simulink library "NREL_Diesel_Genset_lib"  (Simulink 8.1)
settings: Solver=ode45  StartTime=0.0  StopTime=10.0  RelTol=1e-3
values from neighbouring files (symbols this model uses):
  T3dend = [ 1.0000   -0.9913 ]    [initGTS.m]
  T3numd = [ 0    0.0087 ]    [initGTS.m]
  T4numd = [ 27.7778  -27.7237 ]    [initGTS.m]
undefined symbols (not defined in the file or in its folder): DiscIntNeverNeededParam, Efd0, Efd1, Efd2, GP, Ka, Ke, Kf, SeEfd1, SeEfd2, Ta, Te, Tf, Ts, VR0, VRmax, VRmin
libraries: simulink x17, powerlib x9, powerlib_extras x2, powerlib_models x1
(part 1 of 2)
settings Model: Creator=ed12083  LastModifiedBy=pkoralew

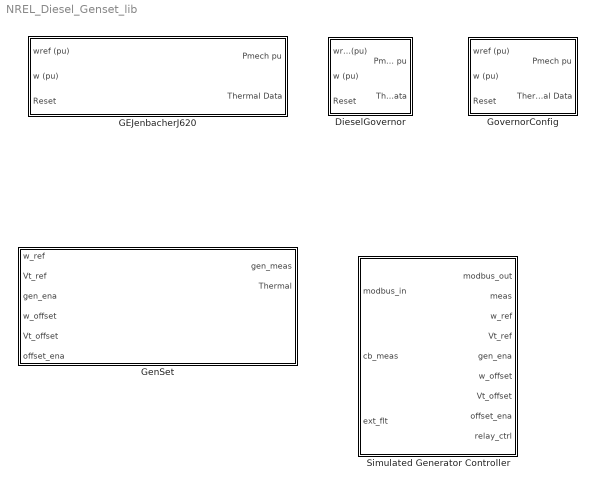
== system NREL_Diesel_Genset_lib ==
  DieselGovernor : Subsystem  mask(Diesel Engine & Governor){K=GP.Gov.Kp, Ta=[0.025 0.0009 0.00574], Tlim=[0 2], Td=0.024, Pm0=0.00005}
      mask prompts: K "Regulator gain K:"; Ta "Actuator time constants [T4 T5 T6] (s) :"; Tlim "Torque limits [Tmin Tmax] (pu) :"; Td "Engine time delay Td (s) :"; Pm0 "Initial value of mechanical power  Pm0 (pu) :"
      mask help:
      | This block implements a diesel engine and governor system:
      | 1st and 2nd inputs: Desired and actual speed (pu)
      | Output: Diesel engine mechanical power.Motor inertia should be combined with generator.
      |
      | Actuator transfer function :
      |      Ha= (1+T4.s) / [ (s (1+T5.s)(1+T6.s) ]
      | Motor :
      |      Time delay Td
      |
      | (See reference in Tutorial Session 5)
  GEJenbacherJ620 : Subsystem  mask{cd=.8, H=47133, keq=1.3962, Ma=.029, Meq=.0285, Mf=.019, P0=800000, Pm=37241, R=8.314, T0=300, Tm=325, thermalEfficiency=.45, V=0.031, Vd=0.125, volumeEfficiency=.9, P=3, I=3, UL=1.05, LL=0, UPL=1.5, LPL=0}
      mask prompts: cd "Discharge coefficient - cd"; H "NG heating value - H"; keq "Equivalent ratio of specific heats of air/fuel mixture - keq"; Ma "Molecular weight of air - Ma"; Meq "Equivalent molecular weight of air/fuel mixture - Meq"; Mf "Molecular weight of NG - Mf"; P0 "Throttle inlet air pressure - P0"; Pm "Intake manifold pressure - Pm"; R "Universal gas constant - R"; T0 "Throttle inlet charge temperature - T0"; Tm "Intake manifold temperature - Tm"; thermalEfficiency "Thermal efficiency - thermalEfficiency"; V "Manifold plus port passage volume - V"; Vd "Engine displacement - Vd"; volumeEfficiency "Volumetric efficiency - volumeEfficiency"; P "Proportional Gain - P"; I "Integral Gain - I"; UL "Upper Integrator Limit - UL"; LL "Lower Integrator Limit - LL"; UPL "Upper Power Limit - UPL"; LPL "Lower Power Limit - LPL"
      mask help: All units are MKS. Refer to "Modeling and Validation of a Lean Burn Natural Gas Engine", Gangopadhyay et. al., ASME 2001
  GenSet : Subsystem  mask{GenSel=3.5MVA natural gas generator}
      mask prompts: GenSel "Generator Preset"
      mask init:
      | GP = initDiesel(GenSel);
      | 
      | dispstr = 'Diesel Generator\n';
      | dispstr = [dispstr 'Pn=' num2str(GP.Pn/1000) ' kW\n'];
      | dispstr = [dispstr 'Vn=' num2str(GP.Vn/1000) ' kV\n'];
      | 
      | govPath = [gcb '/GeneratorWPrimaryControllers/DieselSpeed&Voltage/Governor'];
      | 
      | switch GenSel
      |     case 1
      |         set_param(govPath, 'BlockChoice', 'DieselGovernor');
      |     case 2
      |         set_param(govPath, 'BlockChoice', 'DieselGovernor');
      |     case 3
      |         set_param(govPath, 'BlockChoice', 'DieselGovernor');
      |         %set_param(govPath, 'BlockChoice', 'GEJenbacherJ620');
      | end
      mask TypeOptions GenSel: 4MVA diesel generator | 80kVA diesel generator | 3.5MVA natural gas generator
      mask Display: disp(dispstr);
  GovernorConfig : Subsystem  BlockChoice=DieselGovernor
      settings: TemplateBlock=self  MemberBlocks=DieselGovernor,GEJenbacherJ620
  Simulated Generator Controller : Subsystem  mask{GenSel=80kVA diesel generator}
      mask prompts: GenSel "Generator preset"
      mask init:
      | GP = initGensetCtrl(GenSel);
      | 
      | dispstr = 'Generator controller\n';
      | dispstr = [dispstr 'Pn=' num2str(GP.Pn/1000) ' kW\n'];
      | dispstr = [dispstr 'Vn=' num2str(GP.Vn/1000) ' kV\n'];
      mask TypeOptions GenSel: 4MVA diesel generator | 80kVA diesel generator | 3.5MVA natural gas generator
      mask Display: disp(dispstr);

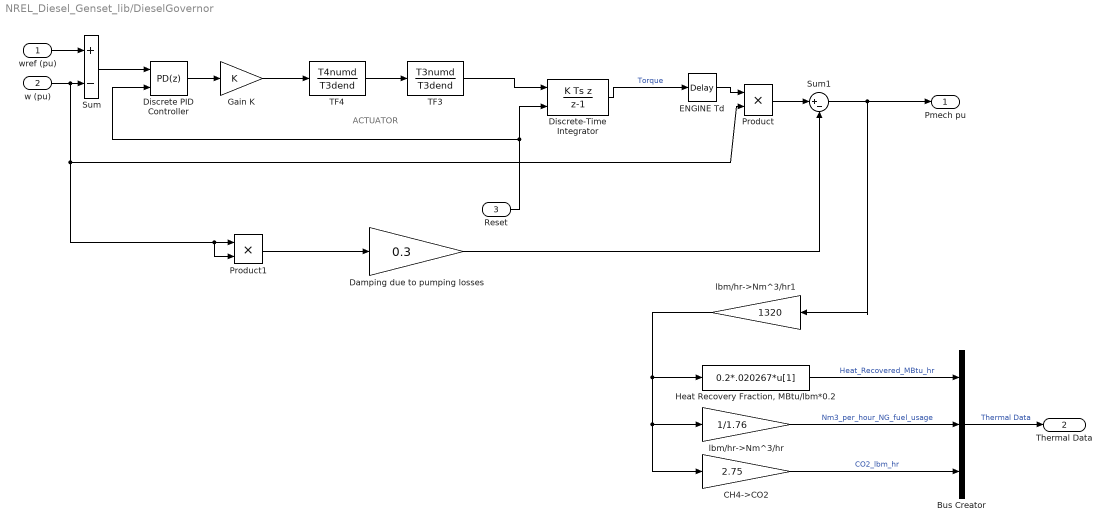
== system NREL_Diesel_Genset_lib/DieselGovernor ==
  note: ACTUATOR
  wref (pu) : Inport
  w (pu) : Inport  Port=2
  Reset : Inport  Port=3
  Bus Creator : BusCreator  Inputs=3
  CH4->CO2 : Gain  Gain=2.75
  Damping due to pumping losses : Gain  Gain=0.3
  Discrete PID Controller : simulink/Continuous/PID Controller  Controller=PD  TimeDomain=Discrete-time  SampleTime=-1  IntegratorMethod=Forward Euler  FilterMethod=Forward Euler  Form=Parallel  P=1  I=0  D=0.5  N=10000  InitialConditionSource=internal  InitialConditionForIntegrator=0  InitialConditionForFilter=0  ExternalReset=level  ZeroCross=off  LimitOutput=off  UpperSaturationLimit=.5  LowerSaturationLimit=-.5  LinearizeAsGain=off  AntiWindupMode=none  Kb=1  TrackingMode=off  Kt=1  PParamMin=[]  PParamMax=[]  IParamMin=[]  IParamMax=[]  DParamMin=[]  DParamMax=[]  NParamMin=[]  NParamMax=[]  KbParamMin=[]  KbParamMax=[]  KtParamMin=[]  KtParamMax=[]  POutMin=[]  POutMax=[]  IOutMin=[]  IOutMax=[]  DOutMin=[]  DOutMax=[]  NOutMin=[]  NOutMax=[]  KbOutMin=[]  KbOutMax=[]  KtOutMin=[]  KtOutMax=[]  IntegratorOutMin=[]  IntegratorOutMax=[]  FilterOutMin=[]  FilterOutMax=[]  SumOutMin=[]  SumOutMax=[]  SumI1OutMin=[]  SumI1OutMax=[]  SumI2OutMin=[]  SumI2OutMax=[]  SumI3OutMin=[]  SumI3OutMax=[]  SumDOutMin=[]  SumDOutMax=[]  SaturationOutMin=[]  SaturationOutMax=[]  IntegratorContinuousStateAttributes=''  IntegratorStateMustResolveToSignalObject=off  IntegratorRTWStateStorageClass=Auto  FilterContinuousStateAttributes=''  FilterStateMustResolveToSignalObject=off  FilterRTWStateStorageClass=Auto
  Discrete-Time Integrator : DiscreteIntegrator  IntegratorMethod=Integration: Backward Euler  ExternalReset=level  InitialCondition=Pm0  SampleTime=-1  LimitOutput=on  UpperSaturationLimit=Tlim(2)  LowerSaturationLimit=Tlim(1)  ICPrevOutput=DiscIntNeverNeededParam  ICPrevScaledInput=DiscIntNeverNeededParam
  ENGINE Td : TransportDelay  DelayTime=Td  InitialOutput=Pm0  BufferSize=7168
  Gain K : Gain  Gain=K  SaturateOnIntegerOverflow=on  OutDataTypeStr=Inherit: Same as input  ParamDataTypeStr=Inherit: Same as input
  "Heat Recovery Fraction, MBtu/lbm*0.2 " : Fcn  Expr=0.2*.020267*u[1]
  Product : Product  SaturateOnIntegerOverflow=on  InputSameDT=on  OutDataTypeStr=Inherit: Same as first input
  Product1 : Product
  Sum : Sum  Inputs=+-  SaturateOnIntegerOverflow=on  InputSameDT=on  OutDataTypeStr=Inherit: Same as first input
  Sum1 : Sum  Inputs=|+-
  TF3 : DiscreteTransferFcn  Numerator=T3numd  Denominator=T3dend  SampleTime=Ts  RndMeth=Nearest
  TF4 : DiscreteTransferFcn  Numerator=T4numd  Denominator=T3dend  SampleTime=Ts
  lbm/hr->Nm^3/hr : Gain  Gain=1/1.76
  lbm/hr->Nm^3/hr1 : Gain  Gain=1320
  Pmech pu : Outport
  Thermal Data : Outport  Port=2
  wires:
  Reset/1 -> Discrete PID Controller/2, Discrete-Time Integrator/2
  TF4/1 -> TF3/1
  TF3/1 -> Discrete-Time Integrator/1
  Discrete-Time Integrator/1 -> ENGINE Td/1  "Torque"
  Product/1 -> Sum1/1
  wref (pu)/1 -> Sum/1
  ENGINE Td/1 -> Product/1
  Gain K/1 -> TF4/1
  Sum/1 -> Discrete PID Controller/1
  Discrete PID Controller/1 -> Gain K/1
  w (pu)/1 -> Sum/2, Product1/1, Product1/2, Product/2
  Product1/1 -> Damping due to pumping losses/1
  Sum1/1 -> Pmech pu/1, lbm/hr->Nm^3/hr1/1
  CH4->CO2/1 -> Bus Creator/3  "CO2_lbm_hr"
  lbm/hr->Nm^3/hr/1 -> Bus Creator/2  "Nm3_per_hour_NG_fuel_usage"
  "Heat Recovery Fraction, MBtu/lbm*0.2 "/1 -> Bus Creator/1  "Heat_Recovered_MBtu_hr"
  Damping due to pumping losses/1 -> Sum1/2
  Bus Creator/1 -> Thermal Data/1  "Thermal Data"
  lbm/hr->Nm^3/hr1/1 -> CH4->CO2/1, lbm/hr->Nm^3/hr/1, "Heat Recovery Fraction, MBtu/lbm*0.2 "/1

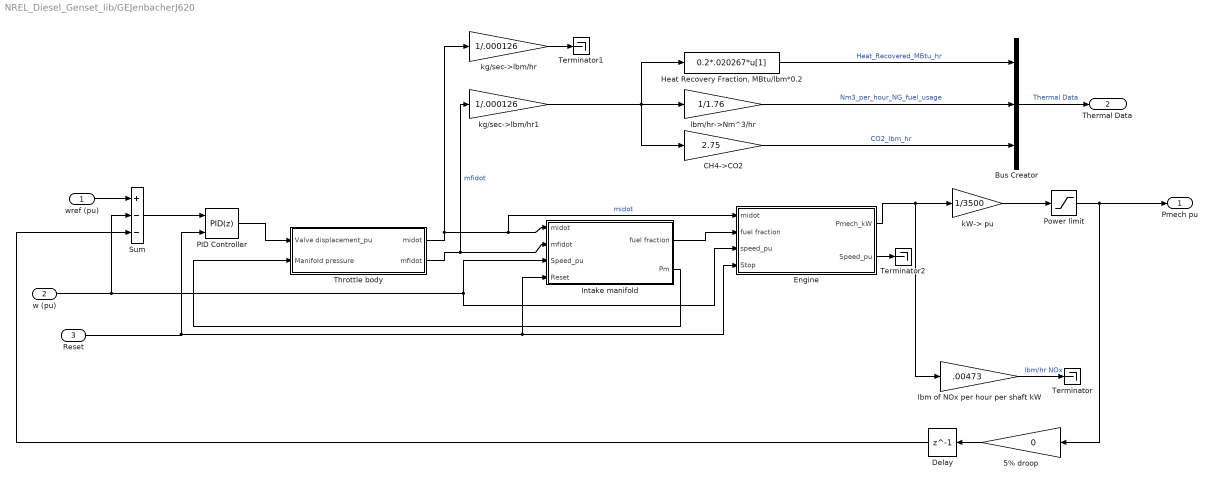
== system NREL_Diesel_Genset_lib/GEJenbacherJ620 ==
  wref (pu) : Inport
  w (pu) : Inport  Port=2
  Reset : Inport  Port=3
  5% droop : Gain  Gain=0
  Bus Creator : BusCreator  Inputs=3
  CH4->CO2 : Gain  Gain=2.75
  Delay : Delay  DelayLength=1  InitialCondition=0
  Engine : Subsystem
  "Heat Recovery Fraction, MBtu/lbm*0.2 " : Fcn  Expr=0.2*.020267*u[1]
  Intake manifold : Subsystem
  PID Controller : simulink/Continuous/PID Controller  Controller=PID  TimeDomain=Discrete-time  SampleTime=Ts  IntegratorMethod=Forward Euler  FilterMethod=Forward Euler  Form=Parallel  P=P  I=I  D=0  N=100  InitialConditionSource=internal  InitialConditionForIntegrator=0  InitialConditionForFilter=0  ExternalReset=level  LimitOutput=off  UpperSaturationLimit=inf  LowerSaturationLimit=-inf  LinearizeAsGain=on  AntiWindupMode=none  Kb=1  TrackingMode=off  Kt=1  PParamMin=[]  PParamMax=[]  IParamMin=[]  IParamMax=[]  DParamMin=[]  DParamMax=[]  NParamMin=[]  NParamMax=[]  KbParamMin=[]  KbParamMax=[]  KtParamMin=[]  KtParamMax=[]  POutMin=[]  POutMax=[]  IOutMin=[]  IOutMax=[]  DOutMin=[]  DOutMax=[]  NOutMin=[]  NOutMax=[]  KbOutMin=[]  KbOutMax=[]  KtOutMin=[]  KtOutMax=[]  IntegratorOutMin=[]  IntegratorOutMax=[]  FilterOutMin=[]  FilterOutMax=[]  SumOutMin=[]  SumOutMax=[]  SumI1OutMin=[]  SumI1OutMax=[]  SumI2OutMin=[]  SumI2OutMax=[]  SumI3OutMin=[]  SumI3OutMax=[]  SumDOutMin=[]  SumDOutMax=[]  SaturationOutMin=[]  SaturationOutMax=[]  IntegratorContinuousStateAttributes=''  IntegratorStateMustResolveToSignalObject=off  IntegratorRTWStateStorageClass=Auto  FilterContinuousStateAttributes=''  FilterStateMustResolveToSignalObject=off  FilterRTWStateStorageClass=Auto
  Power limit : Saturate  UpperLimit=UPL  LowerLimit=LPL
  Sum : Sum  Inputs=+--  SaturateOnIntegerOverflow=on  InputSameDT=on  OutDataTypeStr=Inherit: Same as first input
  Terminator : Terminator
  Terminator1 : Terminator
  Terminator2 : Terminator
  Throttle body : Subsystem
  kW-> pu : Gain  Gain=1/3500
  kg/sec->lbm/hr : Gain  Gain=1/.000126
  kg/sec->lbm/hr1 : Gain  Gain=1/.000126
  lbm of NOx per hour per shaft kW : Gain  Gain=.00473
  lbm/hr->Nm^3/hr : Gain  Gain=1/1.76
  Pmech pu : Outport
  Thermal Data : Outport  Port=2
  wires:
  Power limit/1 -> Pmech pu/1, 5% droop/1
  Sum/1 -> PID Controller/1
  lbm of NOx per hour per shaft kW/1 -> Terminator/1  "lbm/hr NOx"
  CH4->CO2/1 -> Bus Creator/3  "CO2_lbm_hr"
  Delay/1 -> Sum/3
  5% droop/1 -> Delay/1
  Reset/1 -> Intake manifold/4(Reset), Engine/4(Stop), PID Controller/2
  PID Controller/1 -> Throttle body/1(Valve displacement_pu)
  wref (pu)/1 -> Sum/1
  kW-> pu/1 -> Power limit/1
  lbm/hr->Nm^3/hr/1 -> Bus Creator/2  "Nm3_per_hour_NG_fuel_usage"
  "Heat Recovery Fraction, MBtu/lbm*0.2 "/1 -> Bus Creator/1  "Heat_Recovered_MBtu_hr"
  Throttle body/2(mfidot) -> Intake manifold/2(mfidot), kg/sec->lbm/hr1/1  "mfidot"
  kg/sec->lbm/hr1/1 -> "Heat Recovery Fraction, MBtu/lbm*0.2 "/1, lbm/hr->Nm^3/hr/1, CH4->CO2/1
  Engine/1(Pmech_kW) -> kW-> pu/1, lbm of NOx per hour per shaft kW/1
  Throttle body/1(midot) -> Intake manifold/1(midot), Engine/1(midot), kg/sec->lbm/hr/1  "midot"
  Intake manifold/2(Pm) -> Throttle body/2("Manifold pressure ")
  Intake manifold/1(fuel fraction) -> Engine/2(fuel fraction)
  w (pu)/1 -> Intake manifold/3(Speed_pu), Engine/3(speed_pu), Sum/2
  Bus Creator/1 -> Thermal Data/1  "Thermal Data"
  kg/sec->lbm/hr/1 -> Terminator1/1
  Engine/2("Speed_pu ") -> Terminator2/1

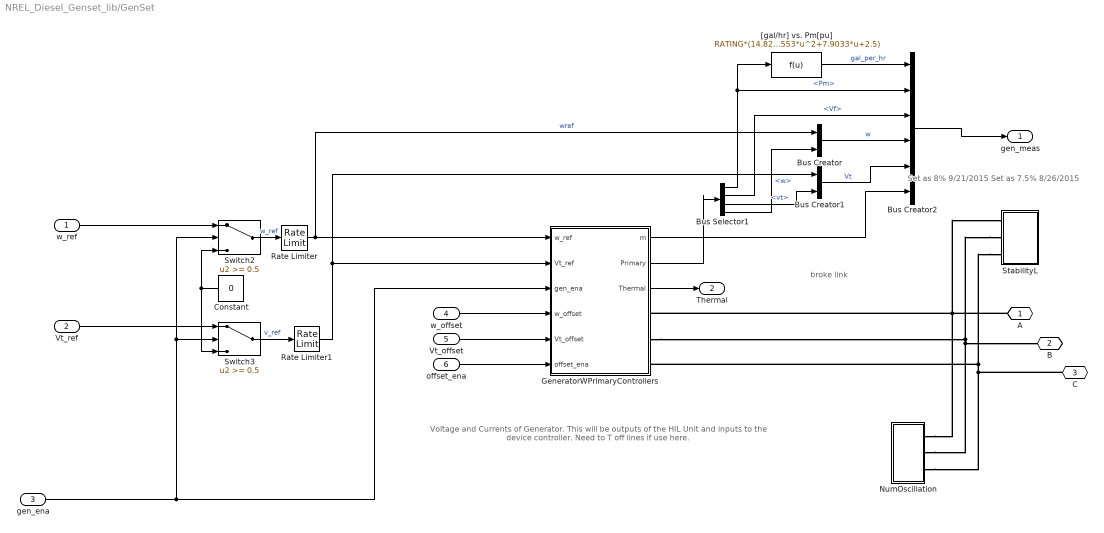
== system NREL_Diesel_Genset_lib/GenSet ==
  note: broke link
  note: Set as 8% 9/21/2015
      | Set as 7.5% 8/26/2015
  note: Voltage and Currents of Generator.
      | This will be outputs of the HIL Unit
      | and inputs to the device controller.
      | Need to T off lines if use here.
  w_ref : Inport
  Vt_ref : Inport  Port=2
  gen_ena : Inport  Port=3
  w_offset : Inport  Port=4
  Vt_offset : Inport  Port=5
  offset_ena : Inport  Port=6
  Bus Creator : BusCreator  Inputs=2
  Bus Creator1 : BusCreator  Inputs=2
  Bus Creator2 : BusCreator  Inputs=6
  Bus Selector1 : BusSelector  OutputSignals=Pm,Vf,vt,w
  Constant : Constant  Value=0
  GeneratorWPrimaryControllers : Subsystem
  NumOscillation : Subsystem
  Rate Limiter : RateLimiter  RisingSlewLimit=0.5  FallingSlewLimit=-0.5  SampleTimeMode=inherited
  Rate Limiter1 : RateLimiter  RisingSlewLimit=0.5  FallingSlewLimit=-0.5  SampleTimeMode=inherited
  StabilityL : Subsystem  mask{v=GP.Vn, kVA=GP.Pn*0.2/1000, pf=1}
  Switch2 : Switch  Threshold=0.5
  Switch3 : Switch  Threshold=0.5
  "[gal/hr] vs. Pm[pu]" : Fcn  Expr=RATING*(14.827*u^4-27.253*u^3+15.553*u^2+7.9033*u+2.5)  mask{RATING=4}
      mask prompts: RATING "Rating [MW]"
      mask help: This block computes the gal/hr vs Pm[pu] of a generator of a given rating [MW].
  A : PMIOPort  Port=1  Side=Right
  B : PMIOPort  Port=2  Side=Right
  C : PMIOPort  Port=3  Side=Right
  gen_meas : Outport
  Thermal : Outport  Port=2
  wires:
  GeneratorWPrimaryControllers/3(Thermal) -> Thermal/1
  "[gal/hr] vs. Pm[pu]"/1 -> Bus Creator2/1  "gal_per_hr"
  Rate Limiter1/1 -> Bus Creator1/1, GeneratorWPrimaryControllers/2(Vt_ref)
  Rate Limiter/1 -> Bus Creator/1, GeneratorWPrimaryControllers/1(w_ref)  "wref"
  Bus Creator2/1 -> gen_meas/1
  Bus Creator/1 -> Bus Creator2/4  "w"
  Bus Creator1/1 -> Bus Creator2/5  "Vt"
  Bus Selector1/1 -> Bus Creator2/2, "[gal/hr] vs. Pm[pu]"/1  "<Pm>"
  Bus Selector1/2 -> Bus Creator2/3  "<Vf>"
  Bus Selector1/4 -> Bus Creator/2  "<w>"
  Bus Selector1/3 -> Bus Creator1/2  "<vt>"
  Switch3/1 -> Rate Limiter1/1  "v_ref"
  Constant/1 -> Switch2/3, Switch3/3
  Switch2/1 -> Rate Limiter/1  "w_ref"
  gen_ena/1 -> Switch3/2, Switch2/2, GeneratorWPrimaryControllers/3(gen_ena)
  GeneratorWPrimaryControllers/2(Primary) -> Bus Selector1/1
  w_ref/1 -> Switch2/1
  w_offset/1 -> GeneratorWPrimaryControllers/4(w_offset)
  Vt_offset/1 -> GeneratorWPrimaryControllers/5(Vt_offset)
  offset_ena/1 -> GeneratorWPrimaryControllers/6(offset_ena)
  Vt_ref/1 -> Switch3/1
  GeneratorWPrimaryControllers/1(m) -> Bus Creator2/6
  connections:
  StabilityL/LConn3 -- GeneratorWPrimaryControllers/RConn3 -- NumOscillation/LConn3 -- C/RConn1
  StabilityL/LConn2 -- B/RConn1 -- NumOscillation/LConn2 -- GeneratorWPrimaryControllers/RConn2
  GeneratorWPrimaryControllers/RConn1 -- StabilityL/LConn1 -- NumOscillation/LConn1 -- A/RConn1

== system NREL_Diesel_Genset_lib/GovernorConfig ==
  wref (pu) : Inport
  w (pu) : Inport  Port=2
  Reset : Inport  Port=3
  DieselGovernor : Subsystem  AncestorBlock=NREL_Diesel_Genset_lib/DieselGovernor  mask(Diesel Engine & Governor){K=GP.Gov.Kp, Ta=[0.025 0.0009 0.00574], Tlim=[0 2], Td=0.024, Pm0=0.00005}
      mask prompts: K "Regulator gain K:"; Ta "Actuator time constants [T4 T5 T6] (s) :"; Tlim "Torque limits [Tmin Tmax] (pu) :"; Td "Engine time delay Td (s) :"; Pm0 "Initial value of mechanical power  Pm0 (pu) :"
      mask help:
      | This block implements a diesel engine and governor system:
      | 1st and 2nd inputs: Desired and actual speed (pu)
      | Output: Diesel engine mechanical power.Motor inertia should be combined with generator.
      |
      | Actuator transfer function :
      |      Ha= (1+T4.s) / [ (s (1+T5.s)(1+T6.s) ]
      | Motor :
      |      Time delay Td
      |
      | (See reference in Tutorial Session 5)
  gnd2 : Ground
  Pmech pu : Outport
  Thermal Data : Outport  Port=2
  wires:
  wref (pu)/1 -> DieselGovernor/1(wref (pu))
  w (pu)/1 -> DieselGovernor/2(w (pu))
  Reset/1 -> DieselGovernor/3(Reset)
  DieselGovernor/1(Pmech pu) -> Pmech pu/1
  gnd2/1 -> Thermal Data/1

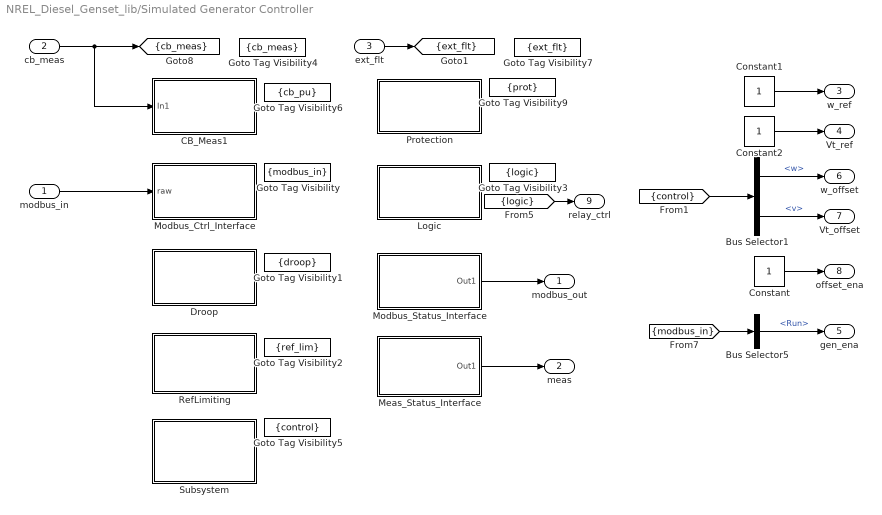
== system NREL_Diesel_Genset_lib/Simulated Generator Controller ==
  modbus_in : Inport
  cb_meas : Inport  Port=2
  ext_flt : Inport  Port=3
  Bus Selector1 : BusSelector  OutputSignals=w,v
  Bus Selector5 : BusSelector  OutputSignals=Control_Word.Run
  CB_Meas1 : Subsystem
  Constant : Constant
  Constant1 : Constant
  Constant2 : Constant
  Droop : Subsystem
  Goto Tag Visibility : GotoTagVisibility  GotoTag=modbus_in
  Goto Tag Visibility1 : GotoTagVisibility  GotoTag=droop
  Goto Tag Visibility2 : GotoTagVisibility  GotoTag=ref_lim
  Goto Tag Visibility3 : GotoTagVisibility  GotoTag=logic
  Goto Tag Visibility4 : GotoTagVisibility  GotoTag=cb_meas
  Goto Tag Visibility5 : GotoTagVisibility  GotoTag=control
  Goto Tag Visibility6 : GotoTagVisibility  GotoTag=cb_pu
  Goto Tag Visibility7 : GotoTagVisibility  GotoTag=ext_flt
  Goto Tag Visibility9 : GotoTagVisibility  GotoTag=prot
  Logic : Subsystem
  Meas_Status_Interface : Subsystem
  Modbus_Ctrl_Interface : Subsystem
  Modbus_Status_Interface : Subsystem
  Protection : Subsystem
  RefLimiting : Subsystem
  Subsystem : Subsystem
  modbus_out : Outport
  meas : Outport  Port=2
  w_ref : Outport  Port=3
  Vt_ref : Outport  Port=4
  gen_ena : Outport  Port=5
  w_offset : Outport  Port=6
  Vt_offset : Outport  Port=7
  offset_ena : Outport  Port=8
  relay_ctrl : Outport  Port=9
  tag scope: cb_meas=scoped, ext_flt=scoped
  wires:
  ext_flt/1 -> [ext_flt]
  Meas_Status_Interface/1(Out1) -> meas/1
  Bus Selector1/2 -> Vt_offset/1  "<v>"
  Bus Selector1/1 -> w_offset/1  "<w>"
  [control] -> Bus Selector1/1
  Bus Selector5/1 -> gen_ena/1  "<Run>"
  [modbus_in] -> Bus Selector5/1
  [logic] -> relay_ctrl/1
  Modbus_Status_Interface/1(Out1) -> modbus_out/1
  cb_meas/1 -> [cb_meas], CB_Meas1/1(In1)
  modbus_in/1 -> Modbus_Ctrl_Interface/1(raw)
  Constant2/1 -> Vt_ref/1
  Constant1/1 -> w_ref/1
  Constant/1 -> offset_ena/1

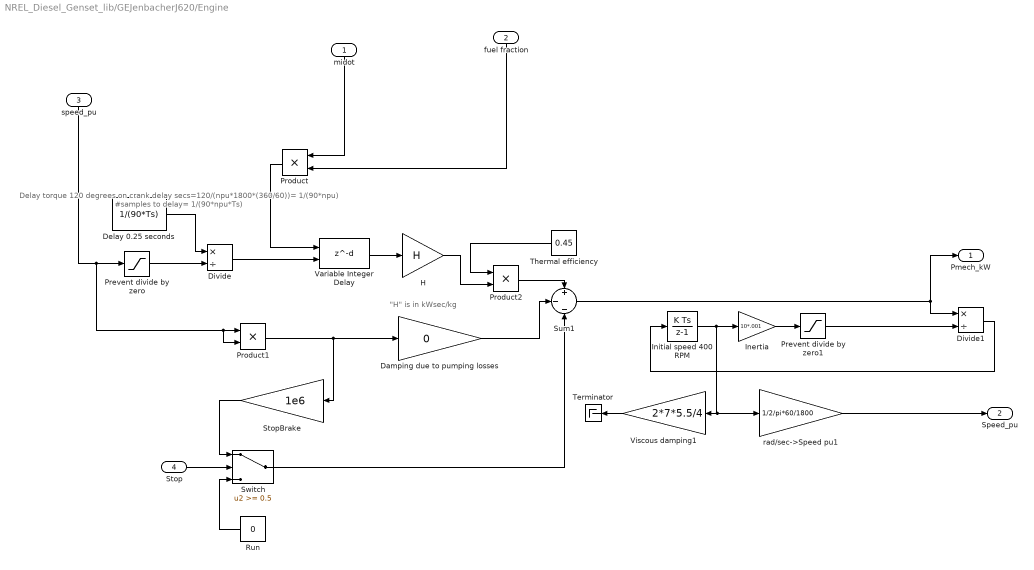
== system NREL_Diesel_Genset_lib/GEJenbacherJ620/Engine ==
  note: Delay torque 120 degrees on crank
      | delay secs=120/(npu*1800*(360/60))= 1/(90*npu)
      | #samples to delay= 1/(90*npu*Ts)
  note: "H" is in kWsec/kg
  midot : Inport
  fuel fraction : Inport  Port=2
  speed_pu : Inport  Port=3
  Stop : Inport  Port=4
  Damping due to pumping losses : Gain  Gain=0
  Delay 0.25 seconds : Constant  Value=1/(90*Ts)
  Divide : Product  Inputs=*/
  Divide1 : Product  Inputs=*/
  H : Gain  Gain=H
  Inertia : Gain  Gain=10*.001
  Initial speed 400 RPM : DiscreteIntegrator  gainval=1  InitialCondition=10/60*2*pi  SampleTime=Ts  LimitOutput=on  LowerSaturationLimit=0  ICPrevOutput=DiscIntNeverNeededParam  ICPrevScaledInput=DiscIntNeverNeededParam
  Prevent divide by zero : Saturate  UpperLimit=inf  LowerLimit=.001
  Prevent divide by zero1 : Saturate  UpperLimit=inf  LowerLimit=.001
  Product : Product
  Product1 : Product
  Product2 : Product
  Run : Constant  Value=0
  StopBrake : Gain  Gain=1e6
  Sum1 : Sum  Inputs=+|-|-
  Switch : Switch  Threshold=0.5
  Terminator : Terminator
  Thermal efficiency : Constant  Value=0.45
  Variable Integer Delay : Delay  DelayLengthSource=Input port  SampleTime=Ts
      settings: InputPortMap=u0,p1
  Viscous damping1 : Gain  Gain=2*7*5.5/4
  rad/sec->Speed pu1 : Gain  Gain=1/2/pi*60/1800
  Pmech_kW : Outport
  "Speed_pu " : Outport  Port=2
  wires:
  StopBrake/1 -> Switch/1
  Run/1 -> Switch/3
  Switch/1 -> Sum1/3
  Stop/1 -> Switch/2
  Damping due to pumping losses/1 -> Sum1/2
  Thermal efficiency/1 -> Product2/1
  Product2/1 -> Sum1/1
  H/1 -> Product2/2
  Prevent divide by zero1/1 -> Divide1/2
  speed_pu/1 -> Product1/2, Product1/1, Prevent divide by zero/1
  Sum1/1 -> Pmech_kW/1, Divide1/1
  rad/sec->Speed pu1/1 -> "Speed_pu "/1
  Divide1/1 -> Initial speed 400 RPM/1
  Inertia/1 -> Prevent divide by zero1/1
  Initial speed 400 RPM/1 -> Inertia/1, rad/sec->Speed pu1/1, Viscous damping1/1
  Divide/1 -> Variable Integer Delay/2
  Delay 0.25 seconds/1 -> Divide/1
  midot/1 -> Product/1
  Prevent divide by zero/1 -> Divide/2
  Variable Integer Delay/1 -> H/1
  Product/1 -> Variable Integer Delay/1
  fuel fraction/1 -> Product/2
  Product1/1 -> Damping due to pumping losses/1, StopBrake/1
  Viscous damping1/1 -> Terminator/1

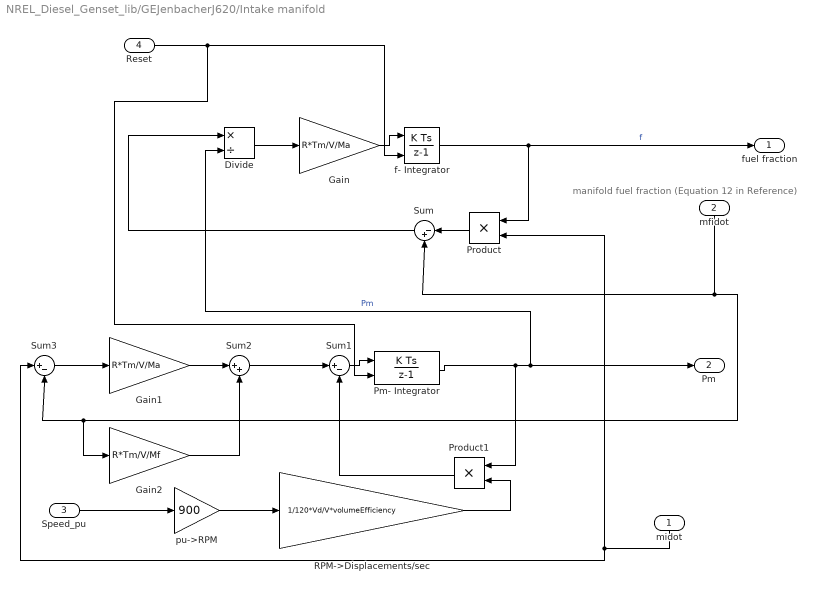
== system NREL_Diesel_Genset_lib/GEJenbacherJ620/Intake manifold ==
  note: manifold fuel fraction
      | (Equation 12 in Reference)
  midot : Inport
  mfidot : Inport  Port=2
  Speed_pu : Inport  Port=3
  Reset : Inport  Port=4
  Divide : Product  Inputs=*/
  Gain : Gain  Gain=R*Tm/V/Ma
  Gain1 : Gain  Gain=R*Tm/V/Ma
  Gain2 : Gain  Gain=R*Tm/V/Mf
  Pm- Integrator : DiscreteIntegrator  ExternalReset=level  InitialCondition=.8/.000145  SampleTime=Ts  LimitOutput=on  UpperSaturationLimit=400000  LowerSaturationLimit=0  ICPrevOutput=DiscIntNeverNeededParam  ICPrevScaledInput=DiscIntNeverNeededParam
  Product : Product
  Product1 : Product
  RPM->Displacements/sec : Gain  Gain=1/120*Vd/V*volumeEfficiency
  Sum : Sum  Inputs=|-+
  Sum1 : Sum  Inputs=|+-
  Sum2 : Sum  Inputs=|++
  Sum3 : Sum  Inputs=|+-
  "f- Integrator " : DiscreteIntegrator  ExternalReset=level  InitialCondition=1/21  SampleTime=Ts  LimitOutput=on  LowerSaturationLimit=0  ICPrevOutput=DiscIntNeverNeededParam  ICPrevScaledInput=DiscIntNeverNeededParam
  pu->RPM : Gain  Gain=900
  fuel fraction : Outport
  Pm : Outport  Port=2
  wires:
  Gain2/1 -> Sum2/2
  Sum3/1 -> Gain1/1
  Sum2/1 -> Sum1/1
  Gain1/1 -> Sum2/1
  mfidot/1 -> Sum3/2, Gain2/1, Sum/2
  RPM->Displacements/sec/1 -> Product1/2
  Product1/1 -> Sum1/2
  midot/1 -> Sum3/1, Product/2
  pu->RPM/1 -> RPM->Displacements/sec/1
  Speed_pu/1 -> pu->RPM/1
  Pm- Integrator/1 -> Product1/1, Pm/1, Divide/2  "Pm"
  Sum1/1 -> Pm- Integrator/1
  Sum/1 -> Divide/1
  Product/1 -> Sum/1
  "f- Integrator "/1 -> Product/1, fuel fraction/1  "f"
  Divide/1 -> Gain/1
  Gain/1 -> "f- Integrator "/1
  Reset/1 -> Pm- Integrator/2, "f- Integrator "/2

== system NREL_Diesel_Genset_lib/GEJenbacherJ620/Throttle body ==
  note: (Equation 1 in Reference)
  note: Total mass flow (air and fuel) into manifold
  note: This subsystem assumes a 2-stage turbocharger supplying boost pressure at 8 bar (800 kPa),
      | valve position in per unit as an independent input, and fixed air/fuel mixture ratio by mass A/F as 20.
      | Manifold pressure is fed back from the intake manifold subsystem
  note: Mass of fuel exiting throttle body into intake manifold
  Valve displacement_pu : Inport
  "Manifold pressure " : Inport  Port=2
  1/P0 : Gain  Gain=1/P0
  A/F=20 : Gain  Gain=1/21
  Force > 0 #2 : Saturate  UpperLimit=inf  LowerLimit=0
  Force > 0 #3 : Saturate  UpperLimit=3  LowerLimit=0
  Product : Product  Inputs=3
  Turbocharger,Throttle,Fuel Mixture #1 : Fcn  Expr=u[1]^(1/keq)*(P0*cd)/sqrt(R/Meq*T0)
  Turbocharger,Throttle,Fuel Mixture #2 : Fcn  Expr=1-u[1]^((keq-1)/keq)
  Turbocharger,Throttle,Fuel Mixture #3 : Fcn  Expr=sqrt(u[1]*(2*keq)/(keq-1))
  Turbocharger,Throttle,Fuel Mixture #4 : Fcn  Expr=0.5*3.7*4.6*(0*2.9e-5+3.2e-5*u[1]+.00034*u[1]^2)
  midot : Outport
  mfidot : Outport  Port=2
  wires:
  1/P0/1 -> Turbocharger,Throttle,Fuel Mixture #1/1, Turbocharger,Throttle,Fuel Mixture #2/1
  Force > 0 #3/1 -> Turbocharger,Throttle,Fuel Mixture #4/1
  Product/1 -> midot/1, A/F=20/1
  Turbocharger,Throttle,Fuel Mixture #4/1 -> Product/3
  Turbocharger,Throttle,Fuel Mixture #3/1 -> Product/2
  Turbocharger,Throttle,Fuel Mixture #1/1 -> Product/1
  Valve displacement_pu/1 -> Force > 0 #3/1
  Force > 0 #2/1 -> Turbocharger,Throttle,Fuel Mixture #3/1
  Turbocharger,Throttle,Fuel Mixture #2/1 -> Force > 0 #2/1
  A/F=20/1 -> mfidot/1
  "Manifold pressure "/1 -> 1/P0/1

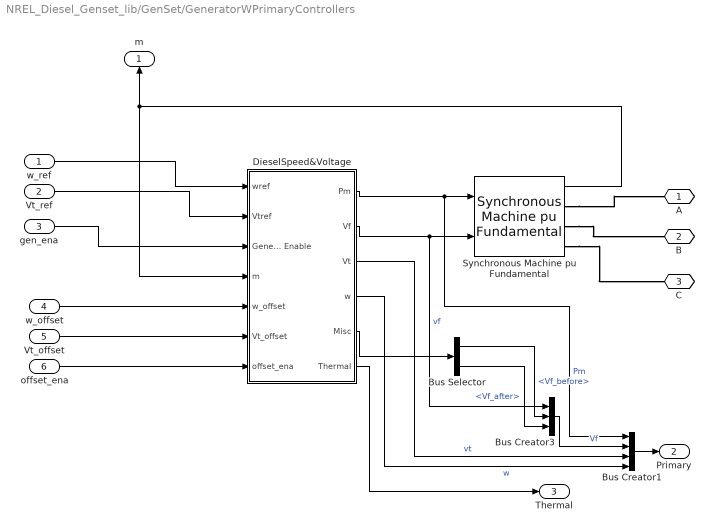
== system NREL_Diesel_Genset_lib/GenSet/GeneratorWPrimaryControllers ==
  w_ref : Inport
  Vt_ref : Inport  Port=2
  gen_ena : Inport  Port=3
  w_offset : Inport  Port=4
  Vt_offset : Inport  Port=5
  offset_ena : Inport  Port=6
  Bus Creator1 : BusCreator
  Bus Creator3 : BusCreator  Inputs=3
  Bus Selector : BusSelector  OutputSignals=Vf_before,Vf_after
  DieselSpeed&Voltage : Subsystem
  Synchronous Machine pu Fundamental : powerlib/Machines/Synchronous Machine pu Fundamental  PresetModel=No  MechanicalLoad=Mechanical power Pm  ShowDetailedParameters=on  RotorType=Salient-pole  NominalParameters=[GP.Pn GP.Vn GP.fn]  Stator=GP.Stator  Field=GP.Field  Dampers2=[0.0652, 0.5134, 0.0287, 0.2553, 7.765e-3, 0.9167 ]  Dampers1=GP.Dampers  Mechanical=GP.Inertia  PolePairs=2  InitialConditions=GP.Initial  SetSaturation=off  Saturation=[0.6404,0.7127,0.8441,0.9214,0.9956,1.082,1.19,1.316,1.457;0.7,0.7698,0.8872,0.9466,0.9969,1.046,1.1,1.151,1.201]  Units=per unit fundamental parameters  LoadFlowParameters=[1,0,0,0,0]  TsPowergui=0  TsBlock=-1  IterativeModel=Trapezoidal non iterative  BusType=swing  Pref=0  Qref=0  Qmin=-inf  Qmax=inf  PLF=0  QLF=0
  A : PMIOPort  Port=1  Side=Right
  B : PMIOPort  Port=2  Side=Right
  C : PMIOPort  Port=3  Side=Right
  m : Outport
  Primary : Outport  Port=2
  Thermal : Outport  Port=3
  wires:
  DieselSpeed&Voltage/6(Thermal) -> Thermal/1
  Bus Creator3/1 -> Bus Creator1/2  "Vf"
  Bus Selector/2 -> Bus Creator3/3  "<Vf_after>"
  Bus Selector/1 -> Bus Creator3/2  "<Vf_before>"
  DieselSpeed&Voltage/5(Misc) -> Bus Selector/1
  Bus Creator1/1 -> Primary/1
  DieselSpeed&Voltage/4(w) -> Bus Creator1/4  "w"
  DieselSpeed&Voltage/3(Vt) -> Bus Creator1/3  "vt"
  Synchronous Machine pu Fundamental/1 -> DieselSpeed&Voltage/4(m), m/1
  gen_ena/1 -> DieselSpeed&Voltage/3(Generator Enable)
  DieselSpeed&Voltage/1(Pm) -> Synchronous Machine pu Fundamental/1, Bus Creator1/1  "Pm"
  DieselSpeed&Voltage/2(Vf) -> Bus Creator3/1, Synchronous Machine pu Fundamental/2  "vf"
  w_ref/1 -> DieselSpeed&Voltage/1(wref)
  Vt_ref/1 -> DieselSpeed&Voltage/2(Vtref)
  w_offset/1 -> DieselSpeed&Voltage/5(w_offset)
  Vt_offset/1 -> DieselSpeed&Voltage/6(Vt_offset)
  offset_ena/1 -> DieselSpeed&Voltage/7(offset_ena)
  connections:
  Synchronous Machine pu Fundamental/RConn1 -- A/RConn1
  Synchronous Machine pu Fundamental/RConn2 -- B/RConn1
  Synchronous Machine pu Fundamental/RConn3 -- C/RConn1

== system NREL_Diesel_Genset_lib/GenSet/NumOscillation ==
  Ground2 : powerlib/Elements/Ground  LConnTagsString=a
  "RLC " : powerlib/Elements/Parallel RLC Branch  LConnTagsString=a  RConnTagsString=__new0  BranchType=R  Resistance=10e6  Inductance=inf  SetiL0=off  InitialCurrent=0  Capacitance=10e-6  Setx0=off  InitialVoltage=0  Measurements=None
  RLC1 : powerlib/Elements/Parallel RLC Branch  LConnTagsString=a  RConnTagsString=__new0  BranchType=R  Resistance=10e6  Inductance=inf  SetiL0=off  InitialCurrent=0  Capacitance=10e-6  Setx0=off  InitialVoltage=0  Measurements=None
  RLC2 : powerlib/Elements/Parallel RLC Branch  LConnTagsString=a  RConnTagsString=__new0  BranchType=R  Resistance=10e6  Inductance=inf  SetiL0=off  InitialCurrent=0  Capacitance=10e-6  Setx0=off  InitialVoltage=0  Measurements=None
  RLC3 : powerlib/Elements/Parallel RLC Branch  LConnTagsString=a  RConnTagsString=__new0  BranchType=R  Resistance=10e-3  Inductance=inf  SetiL0=off  InitialCurrent=0  Capacitance=0  Setx0=off  InitialVoltage=0  Measurements=None
  RLC4 : powerlib/Elements/Parallel RLC Branch  LConnTagsString=a  RConnTagsString=__new0  BranchType=R  Resistance=10e-3  Inductance=inf  SetiL0=off  InitialCurrent=0  Capacitance=0  Setx0=off  InitialVoltage=0  Measurements=None
  RLC5 : powerlib/Elements/Parallel RLC Branch  LConnTagsString=a  RConnTagsString=__new0  BranchType=R  Resistance=10e-3  Inductance=inf  SetiL0=off  InitialCurrent=0  Capacitance=0  Setx0=off  InitialVoltage=0  Measurements=None
  A : PMIOPort  Port=1  Side=Left
  B : PMIOPort  Port=2  Side=Left
  C : PMIOPort  Port=3  Side=Left
  connections:
  "RLC "/RConn1 -- RLC1/RConn1 -- Ground2/LConn1 -- RLC2/RConn1
  "RLC "/LConn1 -- RLC5/RConn1
  RLC1/LConn1 -- RLC4/RConn1
  RLC3/RConn1 -- RLC2/LConn1
  A/RConn1 -- RLC3/LConn1
  B/RConn1 -- RLC4/LConn1
  C/RConn1 -- RLC5/LConn1

== system NREL_Diesel_Genset_lib/GenSet/StabilityL ==
  Constant Load : powerlib/Elements/Three-Phase Parallel RLC Load  LConnTagsString=A|B|C  Configuration=Y (grounded)  NominalVoltage=v  NominalFrequency=60  ActivePower=kVA*1E3*pf  InductivePower=kVA*1E3*sqrt(1-pf^2)  CapacitivePower=0  Measurements=None  LoadType=constant Z
  A : PMIOPort  Port=1  Side=Left
  B : PMIOPort  Port=2  Side=Left
  C : PMIOPort  Port=3  Side=Left
  connections:
  C/RConn1 -- Constant Load/LConn3
  B/RConn1 -- Constant Load/LConn2
  A/RConn1 -- Constant Load/LConn1

== system NREL_Diesel_Genset_lib/GovernorConfig/DieselGovernor ==
  note: ACTUATOR
  wref (pu) : Inport
  w (pu) : Inport  Port=2
  Reset : Inport  Port=3
  Damping due to pumping losses : Gain  Gain=0.3
  Discrete PID Controller : simulink/Continuous/PID Controller  Controller=PD  TimeDomain=Discrete-time  SampleTime=-1  IntegratorMethod=Forward Euler  FilterMethod=Forward Euler  Form=Parallel  P=1  I=0  D=0.5  N=10000  InitialConditionSource=internal  InitialConditionForIntegrator=0  InitialConditionForFilter=0  ExternalReset=level  ZeroCross=off  LimitOutput=off  UpperSaturationLimit=.5  LowerSaturationLimit=-.5  LinearizeAsGain=off  AntiWindupMode=none  Kb=1  TrackingMode=off  Kt=1  PParamMin=[]  PParamMax=[]  IParamMin=[]  IParamMax=[]  DParamMin=[]  DParamMax=[]  NParamMin=[]  NParamMax=[]  KbParamMin=[]  KbParamMax=[]  KtParamMin=[]  KtParamMax=[]  POutMin=[]  POutMax=[]  IOutMin=[]  IOutMax=[]  DOutMin=[]  DOutMax=[]  NOutMin=[]  NOutMax=[]  KbOutMin=[]  KbOutMax=[]  KtOutMin=[]  KtOutMax=[]  IntegratorOutMin=[]  IntegratorOutMax=[]  FilterOutMin=[]  FilterOutMax=[]  SumOutMin=[]  SumOutMax=[]  SumI1OutMin=[]  SumI1OutMax=[]  SumI2OutMin=[]  SumI2OutMax=[]  SumI3OutMin=[]  SumI3OutMax=[]  SumDOutMin=[]  SumDOutMax=[]  SaturationOutMin=[]  SaturationOutMax=[]  IntegratorContinuousStateAttributes=''  IntegratorStateMustResolveToSignalObject=off  IntegratorRTWStateStorageClass=Auto  FilterContinuousStateAttributes=''  FilterStateMustResolveToSignalObject=off  FilterRTWStateStorageClass=Auto
  Discrete-Time Integrator : DiscreteIntegrator  IntegratorMethod=Integration: Backward Euler  ExternalReset=level  InitialCondition=Pm0  SampleTime=-1  LimitOutput=on  UpperSaturationLimit=Tlim(2)  LowerSaturationLimit=Tlim(1)  ICPrevOutput=DiscIntNeverNeededParam  ICPrevScaledInput=DiscIntNeverNeededParam
  ENGINE Td : TransportDelay  DelayTime=Td  InitialOutput=Pm0  BufferSize=7168
  Gain K : Gain  Gain=K  SaturateOnIntegerOverflow=on  OutDataTypeStr=Inherit: Same as input  ParamDataTypeStr=Inherit: Same as input
  Product : Product  SaturateOnIntegerOverflow=on  InputSameDT=on  OutDataTypeStr=Inherit: Same as first input
  Product1 : Product
  Sum : Sum  Inputs=+-  SaturateOnIntegerOverflow=on  InputSameDT=on  OutDataTypeStr=Inherit: Same as first input
  Sum1 : Sum  Inputs=|+-
  TF3 : DiscreteTransferFcn  Numerator=T3numd  Denominator=T3dend  SampleTime=Ts  RndMeth=Nearest
  TF4 : DiscreteTransferFcn  Numerator=T4numd  Denominator=T3dend  SampleTime=Ts
  Pmech pu : Outport
  wires:
  Reset/1 -> Discrete PID Controller/2, Discrete-Time Integrator/2
  TF4/1 -> TF3/1
  TF3/1 -> Discrete-Time Integrator/1
  Discrete-Time Integrator/1 -> ENGINE Td/1  "Torque"
  Product/1 -> Sum1/1
  wref (pu)/1 -> Sum/1
  ENGINE Td/1 -> Product/1
  Gain K/1 -> TF4/1
  Sum/1 -> Discrete PID Controller/1
  Discrete PID Controller/1 -> Gain K/1
  w (pu)/1 -> Sum/2, Product1/1, Product1/2, Product/2
  Damping due to pumping losses/1 -> Sum1/2
  Product1/1 -> Damping due to pumping losses/1
  Sum1/1 -> Pmech pu/1

== system NREL_Diesel_Genset_lib/Simulated Generator Controller/CB_Meas1 ==
  In1 : Inport
  Bus Creator : BusCreator
  Bus Selector : BusSelector  OutputSignals=cb_meas
  Bus Selector1 : BusSelector  OutputSignals=Vabc_line,Iabc
  Bus Selector2 : BusSelector  OutputSignals=relay_out
  Bus Selector3 : BusSelector  OutputSignals=m
  Bus Selector4 : BusSelector  OutputSignals=kw,kvar
  Gain : Gain  Gain=1000/GP.Pn
  Gain1 : Gain  Gain=1000/GP.Pn
  Gain2 : Gain  Gain=1/GP.In/sqrt(2)
  Gain4 : Gain  Gain=1/(GP.Vn*sqrt(2/3))
  tag scope: cb_pu=scoped
  wires:
  Gain1/1 -> Bus Creator/4  "q"
  Gain/1 -> Bus Creator/3  "p"
  In1/1 -> Bus Selector/1, Bus Selector2/1
  Bus Selector4/2 -> Gain1/1  "<kvar>"
  Bus Selector4/1 -> Gain/1  "<kw>"
  Bus Selector3/1 -> Bus Selector4/1  "<m>"
  Bus Selector2/1 -> Bus Selector3/1  "<relay_out>"
  Bus Creator/1 -> [cb_pu]
  Gain2/1 -> Bus Creator/2  "iabc"
  Bus Selector1/2 -> Gain2/1  "<Iabc>"
  Gain4/1 -> Bus Creator/1  "vabc_line"
  Bus Selector1/1 -> Gain4/1  "<Vabc_line>"
  Bus Selector/1 -> Bus Selector1/1  "<cb_meas>"

== system NREL_Diesel_Genset_lib/Simulated Generator Controller/Droop ==
  Bus Selector1 : BusSelector  OutputSignals=relay_out
  Bus Selector3 : BusSelector  OutputSignals=m.Hz,m.Va_rms,m.kw,m.kvar  OutputAsBus=on
  Bus Selector9 : BusSelector  OutputSignals=f_cmd,v_cmd,p_cmd,q_cmd  OutputAsBus=on
  Constant : Constant  Value=[0 0]
  Divide1 : Product  Inputs=*/
  Droop : Subsystem
  ExtractCoefs : Subsystem
  Mux1 : Mux  Inputs=2
  ScalingFactors1 : Constant  Value=[60 GP.Vn/sqrt(3) [1 1]*GP.Pn/1000]
  Selector1 : Selector  InputPortWidth=4  IndexOptions=Index vector (dialog)  Indices=[1 2]  OutputSizes=1
  Sum1 : Sum  Inputs=-+|
  Sum2 : Sum  Inputs=++|
  tag scope: droop=scoped
  wires:
  [modbus_in] -> ExtractCoefs/1(In1)
  ExtractCoefs/1(Out1) -> Droop/2(droop)
  Bus Selector3/1 -> Divide1/1
  Bus Selector1/1 -> Bus Selector3/1  "<relay_out>"
  [cb_meas] -> Bus Selector1/1
  Bus Selector9/1 -> Selector1/1, Sum2/2
  [modbus_in] -> Bus Selector9/1
  Droop/1(dFvpq_out) -> Sum2/1
  Sum1/1 -> Droop/1(dfvpq)
  Selector1/1 -> Mux1/1
  Mux1/1 -> Sum1/2
  Constant/1 -> Mux1/2
  ScalingFactors1/1 -> Divide1/2
  Divide1/1 -> Sum1/1
  Sum2/1 -> [droop]

== system NREL_Diesel_Genset_lib/Simulated Generator Controller/Logic ==
  Bus Selector1 : BusSelector  OutputSignals=Control_Word.Enable
  Bus Selector2 : BusSelector  OutputSignals=Control_Word.Reset
  Bus Selector4 : BusSelector  OutputSignals=auto_reset
  Constant3 : Constant  Value=2
  Constant4 : Constant  Value=0
  Data Type Conversion : DataTypeConversion  OutDataTypeStr=double
  Logical Operator : Logic  Operator=OR  AllPortsSameDT=off  OutDataTypeStr=boolean
  Logical Operator1 : Logic  Operator=NOT  AllPortsSameDT=off  OutDataTypeStr=boolean
  Logical Operator2 : Logic  AllPortsSameDT=off  OutDataTypeStr=boolean
  Mux : Mux  Inputs=3
  Sum : Sum  Inputs=|+-
  tag scope: logic=scoped
  wires:
  Logical Operator2/1 -> Sum/2
  Logical Operator1/1 -> Logical Operator2/2
  [ext_flt] -> Logical Operator1/1
  Data Type Conversion/1 -> Mux/1
  Logical Operator/1 -> Data Type Conversion/1
  Bus Selector2/1 -> Logical Operator/1  "<Reset>"
  [modbus_in] -> Bus Selector2/1
  Bus Selector1/1 -> Logical Operator2/1  "<Enable>"
  [modbus_in] -> Bus Selector1/1
  Bus Selector4/1 -> Logical Operator/2  "<auto_reset>"
  [prot] -> Bus Selector4/1
  Sum/1 -> Mux/2
  Constant3/1 -> Sum/1
  Constant4/1 -> Mux/3
  Mux/1 -> [logic]

== system NREL_Diesel_Genset_lib/Simulated Generator Controller/Meas_Status_Interface ==
  Bus Creator4 : BusCreator  Inputs=2
  Bus Selector : BusSelector  OutputSignals=raw
  Out1 : Outport
  wires:
  Bus Selector/1 -> Bus Creator4/2  "<raw>"
  [modbus_in] -> Bus Selector/1
  [control] -> Bus Creator4/1  "control"
  Bus Creator4/1 -> Out1/1

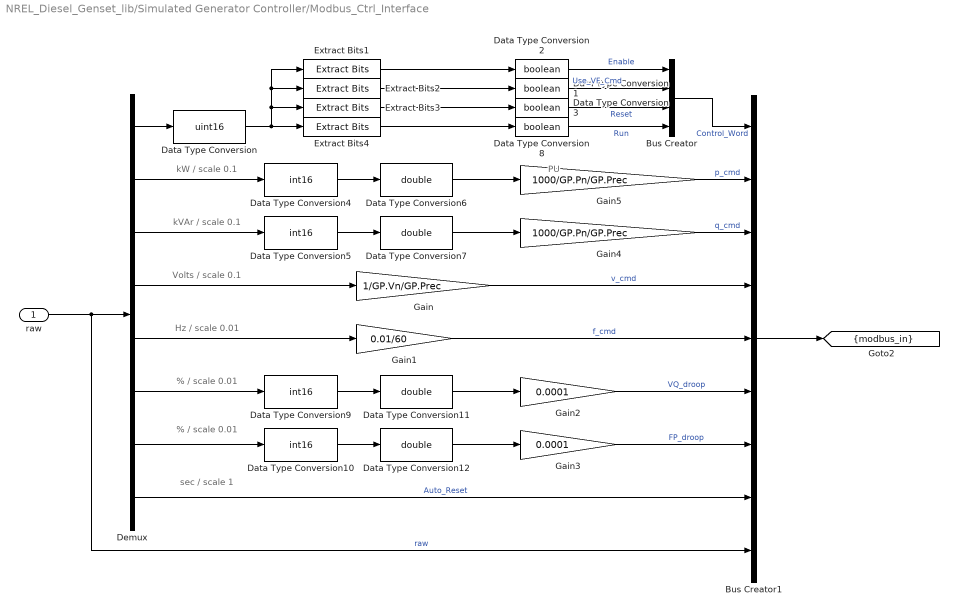
== system NREL_Diesel_Genset_lib/Simulated Generator Controller/Modbus_Ctrl_Interface ==
  note: sec / scale 1
  note: % / scale 0.01
  note: % / scale 0.01
  note: Hz / scale 0.01
  note: Volts / scale 0.1
  note: kVAr / scale 0.1
  note: PU
  note: kW / scale 0.1
  raw : Inport
  Bus Creator : BusCreator
  Bus Creator1 : BusCreator  Inputs=9
  Data Type Conversion : DataTypeConversion  OutDataTypeStr=uint16
  Data Type Conversion{1..3,8} (4 alike) : DataTypeConversion  OutDataTypeStr=boolean
  Data Type Conversion{4..5,9..10} (4 alike) : DataTypeConversion  OutDataTypeStr=int16
  Data Type Conversion{6..7,11..12} (4 alike) : DataTypeConversion  OutDataTypeStr=double
  Demux : Demux  Outputs=8
  Extract Bits1 : simulink/Logic and Bit Operations/Extract Bits  bitsToExtract=Range of bits  numBits=8  bitIdxRange=[0]  outScalingMode=Treat bit field as an integer
  Extract Bits2 : simulink/Logic and Bit Operations/Extract Bits  bitsToExtract=Range of bits  numBits=8  bitIdxRange=[1]  outScalingMode=Treat bit field as an integer
  Extract Bits3 : simulink/Logic and Bit Operations/Extract Bits  bitsToExtract=Range of bits  numBits=8  bitIdxRange=[2]  outScalingMode=Treat bit field as an integer
  Extract Bits4 : simulink/Logic and Bit Operations/Extract Bits  bitsToExtract=Range of bits  numBits=8  bitIdxRange=[3]  outScalingMode=Treat bit field as an integer
  Gain : Gain  Gain=1/GP.Vn/GP.Prec
  Gain1 : Gain  Gain=0.01/60
  Gain2 : Gain  Gain=0.0001
  Gain3 : Gain  Gain=0.0001
  Gain4 : Gain  Gain=1000/GP.Pn/GP.Prec
  Gain5 : Gain  Gain=1000/GP.Pn/GP.Prec
  tag scope: modbus_in=scoped
  wires:
  raw/1 -> Demux/1, Bus Creator1/9  "raw"
  Data Type Conversion12/1 -> Gain3/1
  Data Type Conversion11/1 -> Gain2/1
  Data Type Conversion10/1 -> Data Type Conversion12/1
  Data Type Conversion9/1 -> Data Type Conversion11/1
  Data Type Conversion8/1 -> Bus Creator/4  "Run"
  Extract Bits4/1 -> Data Type Conversion8/1
  Extract Bits2/1 -> Data Type Conversion1/1
  Data Type Conversion7/1 -> Gain4/1
  Data Type Conversion6/1 -> Gain5/1
  Data Type Conversion5/1 -> Data Type Conversion7/1
  Data Type Conversion4/1 -> Data Type Conversion6/1
  Gain5/1 -> Bus Creator1/2  "p_cmd"
  Gain4/1 -> Bus Creator1/3  "q_cmd"
  Demux/2 -> Data Type Conversion4/1
  Data Type Conversion3/1 -> Bus Creator/3  "Reset"
  Data Type Conversion1/1 -> Bus Creator/2  "Use_VF_Cmd"
  Data Type Conversion2/1 -> Bus Creator/1  "Enable"
  Bus Creator1/1 -> [modbus_in]
  Demux/8 -> Bus Creator1/8  "Auto_Reset"
  Gain3/1 -> Bus Creator1/7  "FP_droop"
  Demux/7 -> Data Type Conversion10/1
  Gain2/1 -> Bus Creator1/6  "VQ_droop"
  Demux/6 -> Data Type Conversion9/1
  Gain1/1 -> Bus Creator1/5  "f_cmd"
  Demux/5 -> Gain1/1
  Gain/1 -> Bus Creator1/4  "v_cmd"
  Demux/4 -> Gain/1
  Demux/3 -> Data Type Conversion5/1
  Bus Creator/1 -> Bus Creator1/1  "Control_Word"
  Extract Bits3/1 -> Data Type Conversion3/1
  Extract Bits1/1 -> Data Type Conversion2/1
  Data Type Conversion/1 -> Extract Bits4/1, Extract Bits3/1, Extract Bits2/1, Extract Bits1/1
  Demux/1 -> Data Type Conversion/1

== system NREL_Diesel_Genset_lib/Simulated Generator Controller/Modbus_Status_Interface ==
  Bus Selector : BusSelector  OutputSignals=relay_meas
  Bus Selector1 : BusSelector  OutputSignals=signal1,signal2,signal3,signal4,signal5,signal6,signal7,signal8,signal9,signal10,signal11,signal12,signal13,signal14,signal15,signal16,signal17,signal18,kw,kvar,signal21,signal22,signal23,dF,dV,dWt
  Bus Selector2 : BusSelector  OutputSignals=status,flt_word
  Gain{,1..9} (10 alike) : Gain  Gain=GP.Prec
  Mux : Mux  Inputs=28
  Out1 : Outport
  wires:
  Gain9/1 -> Mux/25
  Bus Selector1/25 -> Gain9/1  "<dV>"
  Bus Selector1/26 -> Mux/26  "<dWt>"
  Bus Selector1/24 -> Mux/24  "<dF>"
  Gain8/1 -> Mux/17
  Gain7/1 -> Mux/15
  Gain6/1 -> Mux/13
  Gain5/1 -> Mux/12
  Gain4/1 -> Mux/11
  Gain3/1 -> Mux/10
  Bus Selector2/1 -> Mux/27  "<status>"
  [prot] -> Bus Selector2/1
  Gain2/1 -> Mux/21
  Gain1/1 -> Mux/20
  Gain/1 -> Mux/19
  Bus Selector2/2 -> Mux/28  "<flt_word>"
  Bus Selector1/23 -> Mux/23  "<signal23>"
  Bus Selector1/22 -> Mux/22  "<signal22>"
  Bus Selector1/21 -> Gain2/1  "<signal21>"
  Bus Selector1/20 -> Gain1/1  "<kvar>"
  Bus Selector1/19 -> Gain/1  "<kw>"
  Bus Selector1/18 -> Mux/18  "<signal18>"
  Bus Selector1/17 -> Gain8/1  "<signal17>"
  Bus Selector1/16 -> Mux/16  "<signal16>"
  Bus Selector1/15 -> Gain7/1  "<signal15>"
  Bus Selector1/14 -> Mux/14  "<signal14>"
  Bus Selector1/13 -> Gain6/1  "<signal13>"
  Bus Selector1/12 -> Gain5/1  "<signal12>"
  Bus Selector1/11 -> Gain4/1  "<signal11>"
  Bus Selector1/10 -> Gain3/1  "<signal10>"
  Bus Selector1/9 -> Mux/9  "<signal9>"
  Bus Selector1/8 -> Mux/8  "<signal8>"
  Bus Selector1/7 -> Mux/7  "<signal7>"
  Bus Selector1/6 -> Mux/6  "<signal6>"
  Bus Selector1/5 -> Mux/5  "<signal5>"
  Bus Selector1/4 -> Mux/4  "<signal4>"
  Bus Selector1/3 -> Mux/3  "<signal3>"
  Bus Selector1/2 -> Mux/2  "<signal2>"
  Bus Selector1/1 -> Mux/1  "<signal1>"
  Bus Selector/1 -> Bus Selector1/1  "<relay_meas>"
  Mux/1 -> Out1/1
  [cb_meas] -> Bus Selector/1

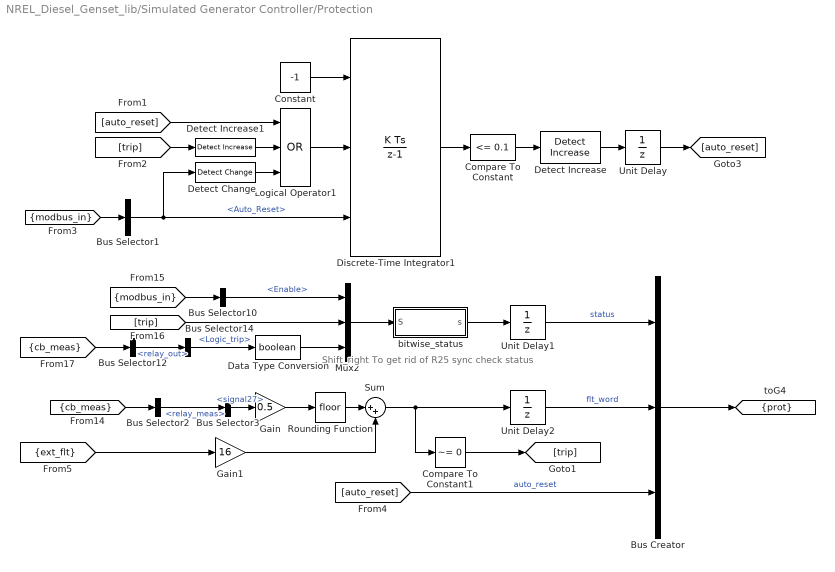
== system NREL_Diesel_Genset_lib/Simulated Generator Controller/Protection ==
  note: Shift_right
      | To get rid of R25 sync check status
  Bus Creator : BusCreator  Inputs=3
  Bus Selector1 : BusSelector  OutputSignals=Auto_Reset
  Bus Selector10 : BusSelector  OutputSignals=Control_Word.Enable
  Bus Selector12 : BusSelector  OutputSignals=relay_out
  Bus Selector14 : BusSelector  OutputSignals=Logic_trip
  Bus Selector2 : BusSelector  OutputSignals=relay_meas
  Bus Selector3 : BusSelector  OutputSignals=signal27
  Compare To Constant : simulink/Logic and Bit Operations/Compare To Constant  relop=<=  const=0.1  OutDataTypeStr=boolean
  Compare To Constant1 : simulink/Logic and Bit Operations/Compare To Constant  relop=~=  const=0  OutDataTypeStr=boolean
  Constant : Constant  Value=-1
  Data Type Conversion : DataTypeConversion  OutDataTypeStr=boolean
  Detect Change : simulink/Logic and Bit Operations/Detect Change  vinit=0  InputProcessing=Inherited  OutDataTypeStr=boolean
  Detect Increase : simulink/Logic and Bit Operations/Detect Increase  vinit=0.0  InputProcessing=Inherited  OutDataTypeStr=boolean
  Detect Increase1 : simulink/Logic and Bit Operations/Detect Increase  vinit=0.0  InputProcessing=Inherited  OutDataTypeStr=boolean
  Discrete-Time Integrator1 : DiscreteIntegrator  ExternalReset=rising  InitialConditionSource=external  SampleTime=Ts  LimitOutput=on  LowerSaturationLimit=0  ICPrevOutput=DiscIntNeverNeededParam  ICPrevScaledInput=DiscIntNeverNeededParam
  Gain : Gain  Gain=0.5
  Gain1 : Gain  Gain=16
  Logical Operator1 : Logic  Operator=OR  Inputs=3  AllPortsSameDT=off  OutDataTypeStr=boolean
  Mux2 : Mux  Inputs=3
  Rounding Function : Rounding
  Sum : Sum  Inputs=|++
  Unit Delay : UnitDelay  SampleTime=-1
  Unit Delay1 : UnitDelay  SampleTime=-1
  Unit Delay2 : UnitDelay  SampleTime=-1
  bitwise_status : Subsystem
  tag scope: prot=scoped
  wires:
  Sum/1 -> Unit Delay2/1, Compare To Constant1/1
  Gain1/1 -> Sum/2
  Rounding Function/1 -> Sum/1
  [ext_flt] -> Gain1/1
  Gain/1 -> Rounding Function/1
  Data Type Conversion/1 -> Mux2/3
  [auto_reset] -> Bus Creator/3  "auto_reset"
  Compare To Constant1/1 -> [trip]
  Bus Selector3/1 -> Gain/1  "<signal27>"
  Bus Selector2/1 -> Bus Selector3/1  "<relay_meas>"
  Unit Delay1/1 -> Bus Creator/1  "status"
  Bus Selector14/1 -> Data Type Conversion/1  "<Logic_trip>"
  Bus Selector12/1 -> Bus Selector14/1  "<relay_out>"
  [cb_meas] -> Bus Selector12/1
  [trip] -> Mux2/2
  Bus Selector10/1 -> Mux2/1  "<Enable>"
  [modbus_in] -> Bus Selector10/1
  Mux2/1 -> bitwise_status/1(S)
  [cb_meas] -> Bus Selector2/1
  Unit Delay2/1 -> Bus Creator/2  "flt_word"
  bitwise_status/1(s) -> Unit Delay1/1
  Detect Change/1 -> Logical Operator1/3
  Bus Selector1/1 -> Discrete-Time Integrator1/3, Detect Change/1  "<Auto_Reset>"
  [modbus_in] -> Bus Selector1/1
  Unit Delay/1 -> [auto_reset]
  Detect Increase/1 -> Unit Delay/1
  Logical Operator1/1 -> Discrete-Time Integrator1/2
  [auto_reset] -> Logical Operator1/1
  Detect Increase1/1 -> Logical Operator1/2
  Compare To Constant/1 -> Detect Increase/1
  Discrete-Time Integrator1/1 -> Compare To Constant/1
  [trip] -> Detect Increase1/1
  Constant/1 -> Discrete-Time Integrator1/1
  Bus Creator/1 -> [prot]

== system NREL_Diesel_Genset_lib/Simulated Generator Controller/RefLimiting ==
  Bus Creator : BusCreator
  Complex to Magnitude-Angle : ComplexToMagnitudeAngle
  Complex to Real-Imag : ComplexToRealImag
  Demux : Demux
  Magnitude-Angle to Complex : MagnitudeAngleToComplex
  Real-Imag to Complex : RealImagToComplex
  Saturation : Saturate  UpperLimit=1.1  LowerLimit=0.9
  Saturation1 : Saturate  UpperLimit=1.1  LowerLimit=0.9
  Saturation2 : Saturate  UpperLimit=1  LowerLimit=0
  tag scope: ref_lim=scoped
  wires:
  Saturation1/1 -> Bus Creator/2  "v"
  Magnitude-Angle to Complex/1 -> Complex to Real-Imag/1
  Bus Creator/1 -> [ref_lim]  "fvpq"
  Demux/3 -> Real-Imag to Complex/1
  Complex to Magnitude-Angle/1 -> Saturation2/1
  Complex to Real-Imag/2 -> Bus Creator/4  "q"
  Complex to Real-Imag/1 -> Bus Creator/3  "p"
  Real-Imag to Complex/1 -> Complex to Magnitude-Angle/1
  Demux/2 -> Saturation1/1
  Demux/1 -> Saturation/1
  [droop] -> Demux/1
  Saturation2/1 -> Magnitude-Angle to Complex/1
  Saturation/1 -> Bus Creator/1  "f"
  Complex to Magnitude-Angle/2 -> Magnitude-Angle to Complex/2
  Demux/4 -> Real-Imag to Complex/2

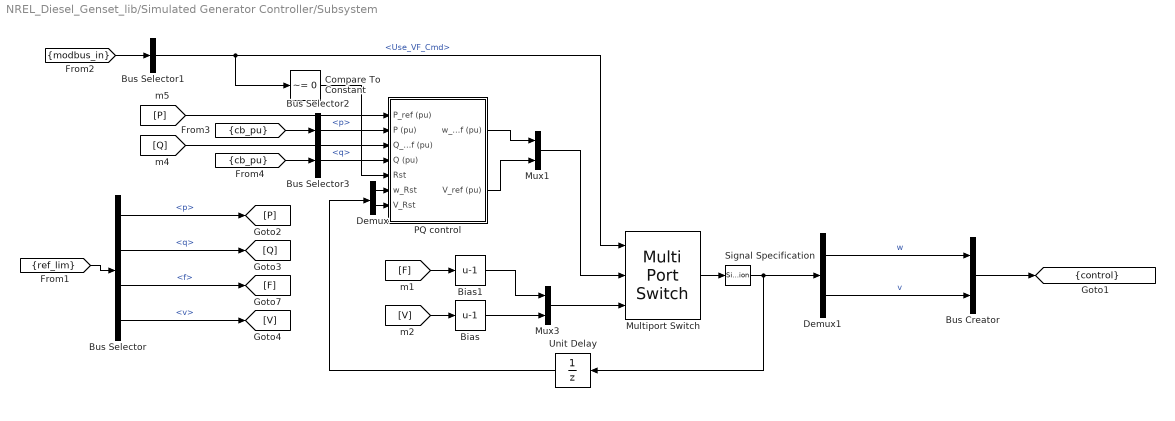
== system NREL_Diesel_Genset_lib/Simulated Generator Controller/Subsystem ==
  Bias : Bias  Bias=-1
  Bias1 : Bias  Bias=-1
  Bus Creator : BusCreator  Inputs=2
  Bus Selector : BusSelector  OutputSignals=p,q,f,v
  Bus Selector1 : BusSelector  OutputSignals=Control_Word.Use_VF_Cmd
  Bus Selector2 : BusSelector  OutputSignals=p
  Bus Selector3 : BusSelector  OutputSignals=q
  Compare To Constant : simulink/Logic and Bit Operations/Compare To Constant  relop=~=  const=0  OutDataTypeStr=boolean
  Demux : Demux  Outputs=2
  Demux1 : Demux  Outputs=[1 1]
  Multiport Switch : MultiPortSwitch  DataPortOrder=Zero-based contiguous  Inputs=2  DiagnosticForDefault=Warning
  Mux1 : Mux  Inputs=2
  Mux3 : Mux  Inputs=2
  PQ control : Subsystem
  Signal Specification : SignalSpecification  Dimensions=2
  Unit Delay : UnitDelay  SampleTime=-1
  tag scope: control=scoped
  wires:
  Bus Creator/1 -> [control]
  Bus Selector2/1 -> PQ control/2(P (pu))  "<p>"
  [Q] -> PQ control/3(Q_ref (pu))
  [cb_pu] -> Bus Selector3/1
  Bus Selector3/1 -> PQ control/4(Q (pu))  "<q>"
  [modbus_in] -> Bus Selector1/1
  Bus Selector/3 -> [F]  "<f>"
  [ref_lim] -> Bus Selector/1
  Demux1/1 -> Bus Creator/1  "w"
  Compare To Constant/1 -> PQ control/5(Rst)
  Bus Selector/1 -> [P]  "<p>"
  Unit Delay/1 -> Demux/1
  Bus Selector/2 -> [Q]  "<q>"
  Bus Selector/4 -> [V]  "<v>"
  Bias1/1 -> Mux3/1
  Demux/1 -> PQ control/6(w_Rst)
  Bias/1 -> Mux3/2
  Mux1/1 -> Multiport Switch/2
  Signal Specification/1 -> Unit Delay/1, Demux1/1
  Multiport Switch/1 -> Signal Specification/1
  Bus Selector1/1 -> Multiport Switch/1, Compare To Constant/1  "<Use_VF_Cmd>"
  [V] -> Bias/1
  Demux1/2 -> Bus Creator/2  "v"
  Demux/2 -> PQ control/7(V_Rst)
  [F] -> Bias1/1
  PQ control/2(V_ref (pu)) -> Mux1/2
  [P] -> PQ control/1(P_ref (pu))
  Mux3/1 -> Multiport Switch/3
  PQ control/1(w_ref (pu)) -> Mux1/1
  [cb_pu] -> Bus Selector2/1
